simulink model "dIPC"  (R2014b)
settings: Solver=ode8  SolverMode=SingleTasking  StartTime=0.0  StopTime=3  FixedStep=1e-3  RelTol=1e-3
values from neighbouring files (symbols this model uses):
  deltav = 500    [DIPCRTinit.m]
  dv = 1500    [DIPCRTinit.m]
  g = [0;0;0]    [DIPCRTinit.m]
  j0 = 0.2    [DIPCRTinit.m]
  j1 = 0.5    [DIPCRTinit.m]
  j2 = 0.5    [DIPCRTinit.m]
  j3 = 0.5    [DIPCRTinit.m]
  j4 = 0.5    [DIPCRTinit.m]
  jv = 0.2    [DIPCRTinit.m]
  kappas = ks/20    (= 6)    [DIPCRTinit.m]
  kappav = 400    [DIPCRTinit.m]
  ks = 120    [DIPCRTinit.m]
  kv = 700    [DIPCRTinit.m]
  m0 = 1.4    [DIPCRTinit.m]
  m1 = 10    [DIPCRTinit.m]
  m2 = 10    [DIPCRTinit.m]
  m3 = 10    [DIPCRTinit.m]
  m4 = 10    [DIPCRTinit.m]
  mv = 1.4    [DIPCRTinit.m]
libraries: aerolibutil x16, dspinverses x3, aerolibtransform2 x2, simulink x2
settings Model: Creator=Martin  LastModifiedBy=Martin
settings OptimizationCC: BlockReduction=off  BooleanDataType=off  UseDivisionForNetSlopeComputation=off  OptimizeBlockIOStorage=off  BufferReuse=off  GlobalBufferReuse=off  ExpressionFolding=off  LocalBlockOutputs=off  SimCompilerOptimization=off
settings DebuggingCC: SaveWithParameterizedLinksMsg=none  UnderspecifiedInitializationDetection=Classic  MergeDetectMultiDrivingBlocksExec=none  SignalResolutionControl=TryResolveAllWithWarning  SolverPrmCheckMsg=none  FrameProcessingCompatibilityMsg=error
settings HardwareCC: TargetUnknown=on
settings RTWCC: RTWCompilerOptimization=off

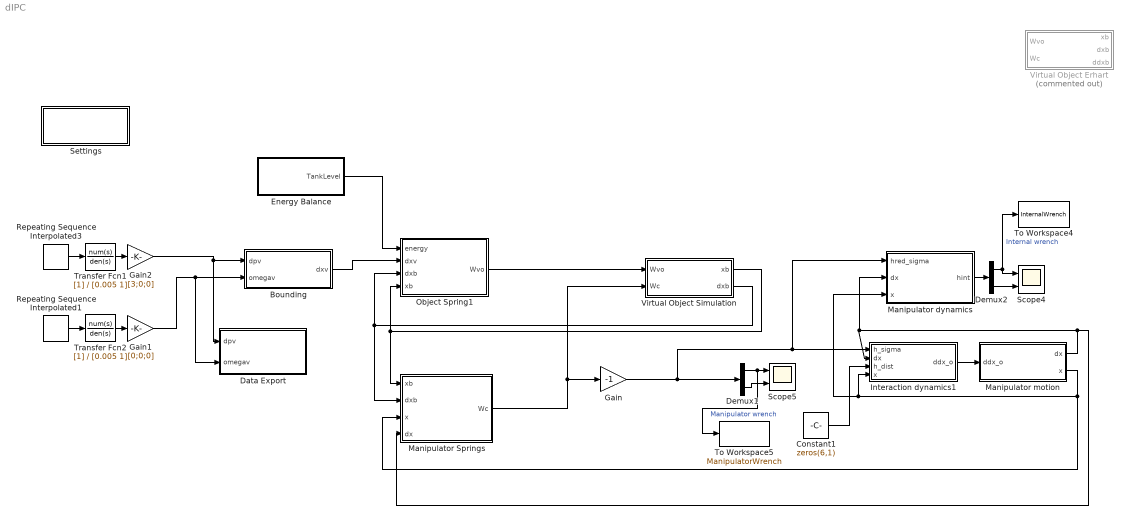
== system dIPC ==
  Bounding : Subsystem
  Constant1 : Constant  Value=zeros(6,1)
  Data Export : Subsystem
  Demux1 : Demux  Outputs=2
  Demux2 : Demux  Outputs=2
  Energy Balance : Subsystem
  Gain : Gain  Gain=-1
  Gain1 : Gain  Gain=[0;0;0]
  Gain2 : Gain  Gain=[3;0;0]
  Interaction dynamics1 : Subsystem
  Manipulator Springs : Subsystem
  Manipulator dynamics : Subsystem
  Manipulator motion : Subsystem
  Object Spring1 : Subsystem
  Repeating Sequence Interpolated1 : simulink/Sources/Repeating Sequence Interpolated  OutValues="[0 0 0.2 0, 0 0.5 0, 0  -0.4 0, 0 0.15 0, 0].'"  TimeValues=[0 0.1 0.25 0.4, 0.6 1 1.5, 1.7 2 2.3, 2.5 2.7 2.9, 3].'  LookUpMeth=Interpolation-Use End Values  tsamp=0.001  OutMin=[]  OutMax=[]  OutDataTypeStr=double  OutputDataTypeScalingMode=double  OutDataType=fixdt(0,8)  OutScaling=2^-10
  Repeating Sequence Interpolated3 : simulink/Sources/Repeating Sequence Interpolated  OutValues="[0 0 0.2 0, 0 0.5 0, 0  -0.4 0, 0 0.15 0, 0].'"  TimeValues=[0 0.1 0.25 0.4, 0.6 1 1.5, 1.7 2 2.3, 2.5 2.7 2.9, 3].'  LookUpMeth=Interpolation-Use End Values  tsamp=0.001  OutMin=[]  OutMax=[]  OutDataTypeStr=double  OutputDataTypeScalingMode=double  OutDataType=fixdt(0,8)  OutScaling=2^-10
  Scope4 : Scope  NumInputPorts=2
      settings: ShowLegends=on  YMin=-0.25~-0.25  YMax=0.25~0.25  SaveName=ScopeData6
  Scope5 : Scope  NumInputPorts=2
      settings: ShowLegends=on  TimeRange=3  YMin=-17.5~-15  YMax=12.5~17.5  SaveName=ScopeData11
  Settings : Subsystem
  To Workspace4 : ToWorkspace  VariableName=InternalWrench  SaveFormat=Timeseries  SampleTime=-1
  To Workspace5 : ToWorkspace  VariableName=ManipulatorWrench  SaveFormat=Timeseries  SampleTime=-1
  Transfer Fcn1 : TransferFcn  Denominator=[0.005 1]
  Transfer Fcn2 : TransferFcn  Denominator=[0.005 1]
  Virtual Object Erhart : Subsystem  Commented=on
  Virtual Object Simulation : Subsystem
  wires:
  Object Spring1/1(Wvo) -> Virtual Object Simulation/1(Wvo)
  Virtual Object Simulation/1(xb) -> Manipulator Springs/1(xb), Object Spring1/4(xb)
  Interaction dynamics1/1(ddx_o) -> Manipulator motion/1(ddx_o)
  Constant1/1 -> Interaction dynamics1/3(h_dist)
  Manipulator motion/2(x) -> Manipulator Springs/3(x), Manipulator dynamics/3(x), Interaction dynamics1/4(x)
  Virtual Object Simulation/2(dxb) -> Manipulator Springs/2(dxb), Object Spring1/3(dxb)
  Manipulator dynamics/1(hint) -> Demux2/1
  Demux2/2 -> Scope4/2
  Demux2/1 -> Scope4/1, To Workspace4/1  "Internal wrench"
  Repeating Sequence Interpolated3/1 -> Transfer Fcn1/1
  Transfer Fcn1/1 -> Gain2/1
  Transfer Fcn2/1 -> Gain1/1
  Demux1/2 -> Scope5/2
  Demux1/1 -> To Workspace5/1, Scope5/1  "Manipulator wrench"
  Gain1/1 -> Data Export/2(omegav), Bounding/2(omegav)
  Gain2/1 -> Data Export/1(dpv), Bounding/1(dpv)
  Bounding/1(dxv) -> Object Spring1/2(dxv)
  Repeating Sequence Interpolated1/1 -> Transfer Fcn2/1
  Manipulator Springs/1(Wc) -> Virtual Object Simulation/2(Wc), Gain/1
  Gain/1 -> Manipulator dynamics/1(hred_sigma), Interaction dynamics1/1(h_sigma), Demux1/1
  Manipulator motion/1(dx) -> Manipulator Springs/4(dx), Manipulator dynamics/2(dx), Interaction dynamics1/2(dx)
  Energy Balance/1(TankLevel) -> Object Spring1/1(energy)

== system dIPC/Bounding ==
  dpv : Inport
  omegav : Inport  Port=2
  Mux : Mux  Inputs=2
  dxv : Outport
  wires:
  dpv/1 -> Mux/1
  omegav/1 -> Mux/2
  Mux/1 -> dxv/1

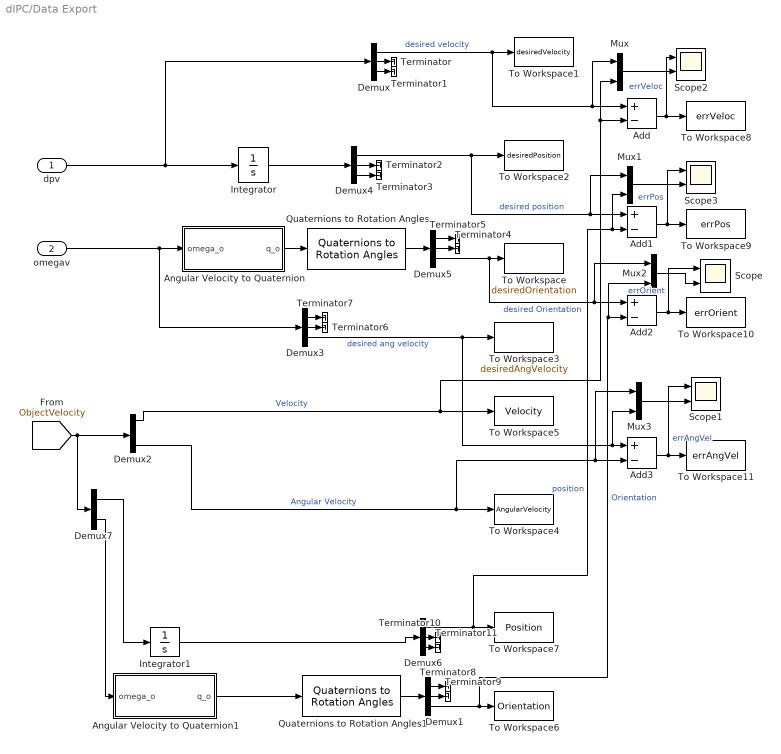
== system dIPC/Data Export ==
  dpv : Inport
  omegav : Inport  Port=2
  Add{,1..3} (4 alike) : Sum  Inputs=+-
  Angular Velocity to Quaternion : Subsystem
  Angular Velocity to Quaternion1 : Subsystem
  Demux{,1,3..6} (6 alike) : Demux  Outputs=3
  Demux2 : Demux  Outputs=6
  Demux7 : Demux  Outputs=2
  Integrator : Integrator
  Integrator1 : Integrator  InitialCondition=[0 0 0]'
  Mux{,1..3} (4 alike) : Mux  Inputs=2
  Quaternions to Rotation Angles : aerolibtransform2/Quaternions to Rotation Angles  rotationOrder=XYZ
  Quaternions to Rotation Angles1 : aerolibtransform2/Quaternions to Rotation Angles  rotationOrder=XYZ
  Scope{,1..3} (4 alike) : Scope  NumInputPorts=2
      Scope settings: YMin=-0.03~-0  YMax=0.035~0.275  SaveName=ScopeData13
      Scope1 settings: ShowLegends=on  YMin=-0.1~-0.4  YMax=0.1~0.6  SaveName=ScopeData37
      Scope2 settings: ShowLegends=on  TimeRange=3  YMin=-0.6~-1.5  YMax=0.6~1.5  SaveName=ScopeData19
      Scope3 settings: YMin=-0.0025~0  YMax=0.03~0.13  SaveName=ScopeData39
  Terminator{,1..11} (12 alike) : Terminator
  To Workspace : ToWorkspace  VariableName=desiredOrientation  SaveFormat=Timeseries  SampleTime=-1
  To Workspace1 : ToWorkspace  VariableName=desiredVelocity  SaveFormat=Timeseries  SampleTime=-1
  To Workspace10 : ToWorkspace  VariableName=errOrient  SaveFormat=Timeseries  SampleTime=-1
  To Workspace11 : ToWorkspace  VariableName=errAngVel  SaveFormat=Timeseries  SampleTime=-1
  To Workspace2 : ToWorkspace  VariableName=desiredPosition  SaveFormat=Timeseries  SampleTime=-1
  To Workspace3 : ToWorkspace  VariableName=desiredAngVelocity  SaveFormat=Timeseries  SampleTime=-1
  To Workspace4 : ToWorkspace  VariableName=AngularVelocity  SaveFormat=Timeseries  SampleTime=-1
  To Workspace5 : ToWorkspace  VariableName=Velocity  SaveFormat=Timeseries  SampleTime=-1
  To Workspace6 : ToWorkspace  VariableName=Orientation  SaveFormat=Timeseries  SampleTime=-1
  To Workspace7 : ToWorkspace  VariableName=Position  SaveFormat=Timeseries  SampleTime=-1
  To Workspace8 : ToWorkspace  VariableName=errVeloc  SaveFormat=Timeseries  SampleTime=-1
  To Workspace9 : ToWorkspace  VariableName=errPos  SaveFormat=Timeseries  SampleTime=-1
  wires:
  Demux4/1 -> Mux1/1, Add1/1, To Workspace2/1  "desired position"
  Demux/1 -> Mux/1, Add/1, To Workspace1/1  "desired velocity"
  Integrator/1 -> Demux4/1
  dpv/1 -> Demux/1, Integrator/1
  Demux/2 -> Terminator/1
  Demux/3 -> Terminator1/1
  Demux4/2 -> Terminator2/1
  Demux4/3 -> Terminator3/1
  Quaternions to Rotation Angles/1 -> Demux5/1
  Demux5/3 -> Mux2/1, Add2/1, To Workspace/1  "desired Orientation"
  Demux3/3 -> Mux3/2, Add3/1, To Workspace3/1  "desired ang velocity"
  Angular Velocity to Quaternion/1(q_o) -> Quaternions to Rotation Angles/1
  omegav/1 -> Demux3/1, Angular Velocity to Quaternion/1(omega_o)
  Demux5/2 -> Terminator4/1
  Demux5/1 -> Terminator5/1
  Demux3/2 -> Terminator6/1
  Demux3/1 -> Terminator7/1
  Demux2/1 -> Mux/2, Add/2, To Workspace5/1  "Velocity"
  Demux2/6 -> Mux3/1, Add3/2, To Workspace4/1  "Angular Velocity"
  [ObjectVelocity] -> Demux7/1, Demux2/1
  Quaternions to Rotation Angles1/1 -> Demux1/1
  Demux1/3 -> Mux2/2, Add2/2, To Workspace6/1  "Orientation"
  Demux1/2 -> Terminator9/1
  Demux1/1 -> Terminator8/1
  Demux6/1 -> Mux1/2, Add1/2, To Workspace7/1  "position"
  Demux6/2 -> Terminator10/1
  Demux6/3 -> Terminator11/1
  Demux7/1 -> Integrator1/1
  Integrator1/1 -> Demux6/1
  Demux7/2 -> Angular Velocity to Quaternion1/1(omega_o)
  Angular Velocity to Quaternion1/1(q_o) -> Quaternions to Rotation Angles1/1
  Add/1 -> Scope2/1, To Workspace8/1  "errVeloc"
  Add1/1 -> Scope3/1, To Workspace9/1  "errPos"
  Add2/1 -> Scope/1, To Workspace10/1  "errOrient"
  Add3/1 -> Scope1/1, To Workspace11/1  "errAngVel"
  Mux/1 -> Scope2/2
  Mux1/1 -> Scope3/2
  Mux2/1 -> Scope/2
  Mux3/1 -> Scope1/2

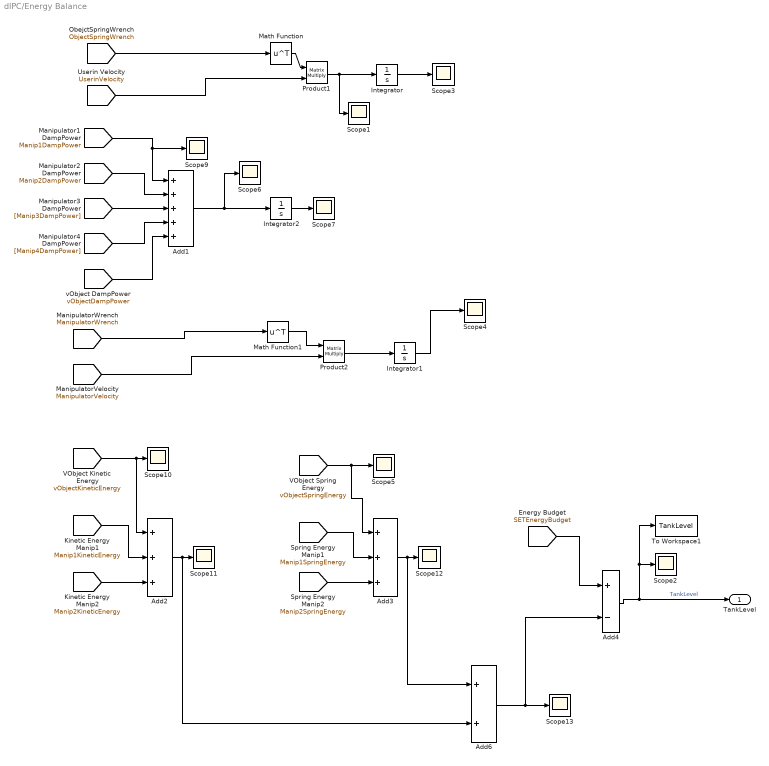
== system dIPC/Energy Balance ==
  Add1 : Sum  Inputs=+++++
  Add2 : Sum  Inputs=+++
  Add3 : Sum  Inputs=+++
  Add4 : Sum  Inputs=+-
  Add6 : Sum
  Integrator : Integrator
  Integrator1 : Integrator
  Integrator2 : Integrator
  Math Function : Math  Operator=transpose  SaturateOnIntegerOverflow=on
  Math Function1 : Math  Operator=transpose  SaturateOnIntegerOverflow=on
  Product1 : Product  Multiplication=Matrix(*)
  Product2 : Product  Multiplication=Matrix(*)
  Scope{1..7,9..13} (12 alike) : Scope
      Scope1 settings: YMin=0  YMax=60  SaveName=ScopeData5
      Scope10 settings: YMin=0  YMax=0.5  SaveName=ScopeData3
      Scope11 settings: YMin=0  YMax=25  SaveName=ScopeData23
      Scope12 settings: YMin=0  YMax=0.6  SaveName=ScopeData36
      Scope13 settings: YMin=1  YMax=9  SaveName=ScopeData38
      Scope2 settings: TimeRange=4.999  YMin=0  YMax=10
      Scope3 settings: TimeRange=5  YMin=0  YMax=12  SaveName=ScopeData14
      Scope4 settings: YMin=-60  YMax=10  SaveName=ScopeData12
      Scope5 settings: YMin=-4.16334e-17  YMax=0.575  SaveName=ScopeData42
      Scope6 settings: YMin=-0.3  YMax=0.05  SaveName=ScopeData40
      Scope7 settings: YMin=675  YMax=1000  SaveName=ScopeData41
      Scope9 settings: YMin=0  YMax=3e-05  SaveName=ScopeData46
  To Workspace1 : ToWorkspace  VariableName=TankLevel  SaveFormat=Timeseries  SampleTime=-1
  TankLevel : Outport
  wires:
  Add4/1 -> TankLevel/1, To Workspace1/1, Scope2/1  "TankLevel"
  Product1/1 -> Integrator/1, Scope1/1
  [UserinVelocity] -> Product1/2
  Integrator/1 -> Scope3/1
  [Manip1DampPower] -> Scope9/1, Add1/1
  [Manip2DampPower] -> Add1/2
  [Manip3DampPower] -> Add1/3
  [Manip4DampPower] -> Add1/4
  [vObjectDampPower] -> Add1/5
  Add1/1 -> Integrator2/1, Scope6/1
  Integrator2/1 -> Scope7/1
  Math Function/1 -> Product1/1
  [ObjectSpringWrench] -> Math Function/1
  Add6/1 -> Add4/2, Scope13/1
  Product2/1 -> Integrator1/1
  Math Function1/1 -> Product2/1
  [ManipulatorVelocity] -> Product2/2
  [ManipulatorWrench] -> Math Function1/1
  Integrator1/1 -> Scope4/1
  [SETEnergyBudget] -> Add4/1
  [vObjectSpringEnergy] -> Scope5/1, Add3/1
  [vObjectKineticEnergy] -> Add2/1, Scope10/1
  Add2/1 -> Add6/2, Scope11/1
  Add3/1 -> Add6/1, Scope12/1
  [Manip2SpringEnergy] -> Add3/3
  [Manip1SpringEnergy] -> Add3/2
  [Manip2KineticEnergy] -> Add2/3
  [Manip1KineticEnergy] -> Add2/2

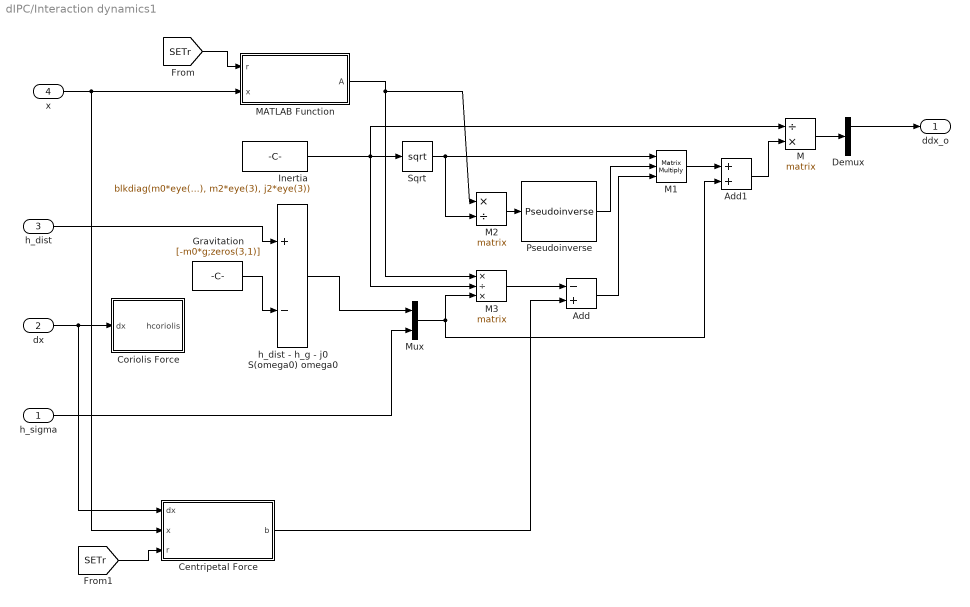
== system dIPC/Interaction dynamics1 ==
  h_sigma : Inport
  dx : Inport  Port=2
  h_dist : Inport  Port=3
  x : Inport  Port=4
  Add : Sum  Inputs=-+
  Add1 : Sum
  Centripetal Force : MATLAB Function  TreatAsAtomicUnit=on
  Coriolis Force : MATLAB Function  TreatAsAtomicUnit=on
  Demux : Demux  Outputs=3
  Gravitation : Constant  Value=[-m0*g;zeros(3,1)]
  Inertia : Constant  Value=blkdiag(m0*eye(3),j0*eye(3),m1*eye(3), j1*eye(3), m2*eye(3), j2*eye(3))
  M : Product  Inputs=/*  Multiplication=Matrix(*)
  M1 : Product  Inputs=***  Multiplication=Matrix(*)
  M2 : Product  Inputs=*/  Multiplication=Matrix(*)
  M3 : Product  Inputs=*/*  Multiplication=Matrix(*)
  MATLAB Function : MATLAB Function  TreatAsAtomicUnit=on
  Mux : Mux  Inputs=2
  Pseudoinverse : dspinverses/Pseudoinverse  wanterr=off
  Sqrt : Sqrt  SaturateOnIntegerOverflow=on
  "h_dist - h_g - j0 S(omega0) omega0 " : Sum  Inputs=+-
  ddx_o : Outport
  wires:
  h_dist/1 -> "h_dist - h_g - j0 S(omega0) omega0 "/1
  Gravitation/1 -> "h_dist - h_g - j0 S(omega0) omega0 "/2
  dx/1 -> Centripetal Force/1(dx), Coriolis Force/1(dx)
  x/1 -> MATLAB Function/2(x), Centripetal Force/2(x)
  Inertia/1 -> M/1, M3/2, Sqrt/1
  Sqrt/1 -> M2/2, M1/1
  MATLAB Function/1(A) -> M3/1, M2/1
  M2/1 -> Pseudoinverse/1
  Pseudoinverse/1 -> M1/2
  Add/1 -> M1/3
  Centripetal Force/1(b) -> Add/2
  M3/1 -> Add/1
  Mux/1 -> Add1/2, M3/3
  "h_dist - h_g - j0 S(omega0) omega0 "/1 -> Mux/1
  h_sigma/1 -> Mux/2
  M/1 -> Demux/1
  Demux/1 -> ddx_o/1
  M1/1 -> Add1/1
  Add1/1 -> M/2
  [SETr] -> MATLAB Function/1(r)
  [SETr] -> Centripetal Force/3(r)

== system dIPC/Manipulator Springs ==
  xb : Inport
  dxb : Inport  Port=2
  x : Inport  Port=3
  dx : Inport  Port=4
  Demux1 : Demux  Outputs=2
  Demux2 : Demux  Outputs=2
  Demux3 : Demux  Outputs=2
  Grasp Matrix : MATLAB Function  TreatAsAtomicUnit=on
  Math Function : Math  Operator=transpose  SaturateOnIntegerOverflow=on
  Mux : Mux  Inputs=2
  Product : Product  Multiplication=Matrix(*)
  Spring 1 : Subsystem
  Spring 2 : Subsystem
  Wc : Outport
  tag scope: ManipulatorWrench=global
  wires:
  Spring 2/1(Wc2) -> Mux/2
  Mux/1 -> [ManipulatorWrench], Wc/1
  Grasp Matrix/1(G) -> Math Function/1
  Math Function/1 -> Product/1
  dxb/1 -> Product/2
  Product/1 -> Demux3/1
  xb/1 -> Spring 1/1(xb), Spring 2/1(xb), Grasp Matrix/1(x)
  Demux3/2 -> Spring 2/2(dxb2)
  Demux3/1 -> Spring 1/2(dxb1)
  Spring 1/1(Wc1) -> Mux/1
  Demux2/1 -> Spring 1/3(x1)
  Demux2/2 -> Spring 2/3(x2)
  Demux1/1 -> Spring 1/4(dx1)
  Demux1/2 -> Spring 2/4(dx2)
  dx/1 -> Demux1/1
  x/1 -> Demux2/1
  [SETrv] -> Grasp Matrix/2(rv)

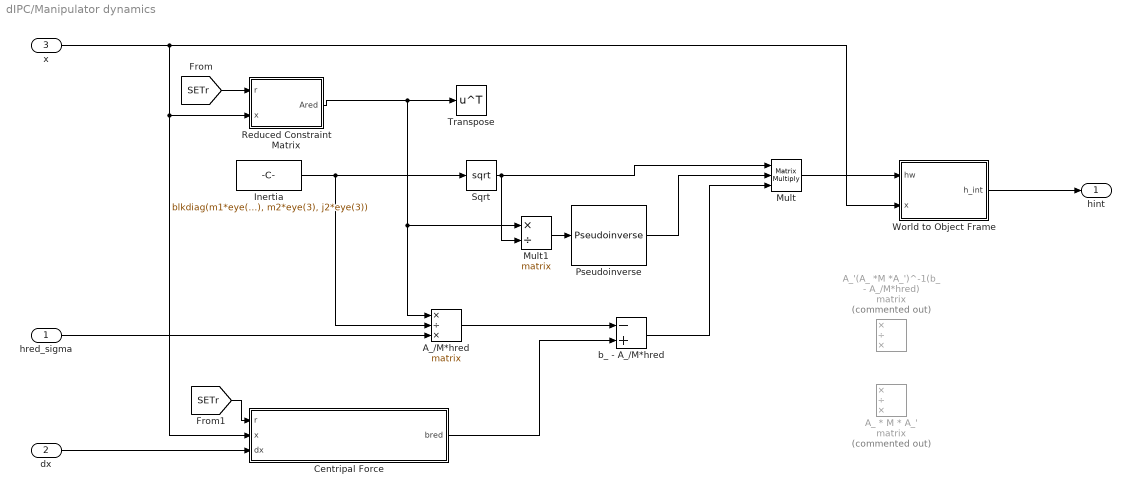
== system dIPC/Manipulator dynamics ==
  hred_sigma : Inport
  dx : Inport  Port=2
  x : Inport  Port=3
  A_ * M * A_' : Product  Commented=on  Inputs=*/*  Multiplication=Matrix(*)
  A_'(A_ *M *A_')^-1(b_ - A_/M*hred) : Product  Commented=on  Inputs=*/*  Multiplication=Matrix(*)
  A_/M*hred : Product  Inputs=*/*  Multiplication=Matrix(*)
  Centripal Force : MATLAB Function  TreatAsAtomicUnit=on
  Inertia : Constant  Value=blkdiag(m1*eye(3), j1*eye(3), m2*eye(3), j2*eye(3))
  Mult : Product  Inputs=***  Multiplication=Matrix(*)
  Mult1 : Product  Inputs=*/  Multiplication=Matrix(*)
  Pseudoinverse : dspinverses/Pseudoinverse  wanterr=off
  Reduced Constraint Matrix : MATLAB Function  TreatAsAtomicUnit=on
  Sqrt : Sqrt  SaturateOnIntegerOverflow=on
  Transpose : Math  Operator=transpose  SaturateOnIntegerOverflow=on
  World to Object Frame : MATLAB Function  TreatAsAtomicUnit=on
  b_ - A_/M*hred : Sum  Inputs=-+
  hint : Outport
  wires:
  Reduced Constraint Matrix/1(Ared) -> Transpose/1, A_/M*hred/1, Mult1/1
  Inertia/1 -> Sqrt/1, A_/M*hred/2
  dx/1 -> Centripal Force/3(dx)
  A_/M*hred/1 -> b_ - A_/M*hred/1
  hred_sigma/1 -> A_/M*hred/3
  World to Object Frame/1(h_int) -> hint/1
  x/1 -> Centripal Force/2(x), Reduced Constraint Matrix/2(x), World to Object Frame/2(x)
  Centripal Force/1(bred) -> b_ - A_/M*hred/2
  Mult/1 -> World to Object Frame/1(hw)
  b_ - A_/M*hred/1 -> Mult/3
  Sqrt/1 -> Mult1/2, Mult/1
  Mult1/1 -> Pseudoinverse/1
  Pseudoinverse/1 -> Mult/2
  [SETr] -> Reduced Constraint Matrix/1(r)
  [SETr] -> Centripal Force/1(r)

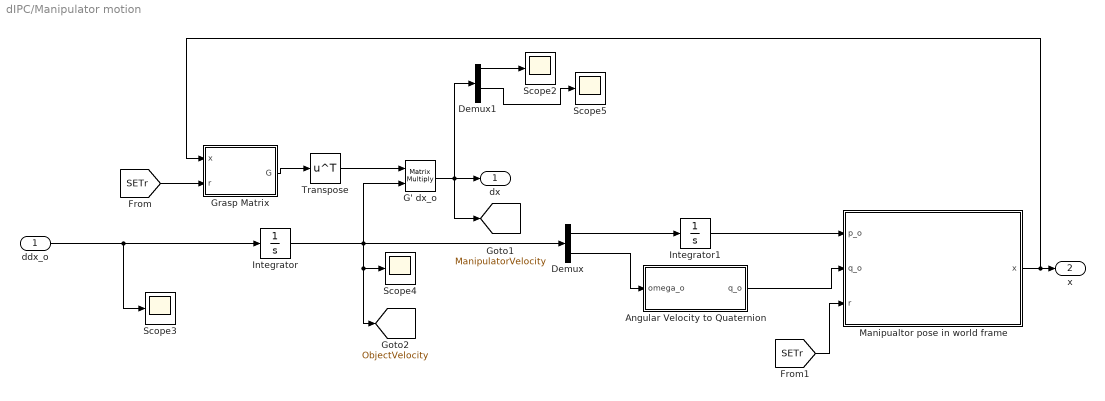
== system dIPC/Manipulator motion ==
  ddx_o : Inport
  Angular Velocity to Quaternion : Subsystem
  Demux : Demux  Outputs=2
  Demux1 : Demux
  G' dx_o : Product  Multiplication=Matrix(*)
  Grasp Matrix : MATLAB Function  TreatAsAtomicUnit=on
  Integrator : Integrator  InitialCondition=zeros(6,1)
  Integrator1 : Integrator  InitialCondition=[0 0 0]'
  Manipualtor pose in world frame : MATLAB Function  TreatAsAtomicUnit=on
  Scope{2..5} (4 alike) : Scope
      Scope2 settings: YMin=-0.02  YMax=0.16  SaveName=ScopeData12
      Scope3 settings: SaveName=ScopeData7
      Scope4 settings: SaveName=ScopeData16
      Scope5 settings: ShowLegends=on  YMin=-0.4  YMax=0.5  SaveName=ScopeData40
  Transpose : Math  Operator=transpose  SaturateOnIntegerOverflow=on
  dx : Outport
  x : Outport  Port=2
  tag scope: ManipulatorVelocity=global, ObjectVelocity=global
  wires:
  ddx_o/1 -> Scope3/1, Integrator/1
  Integrator/1 -> Scope4/1, [ObjectVelocity], G' dx_o/2, Demux/1
  Grasp Matrix/1(G) -> Transpose/1
  Transpose/1 -> G' dx_o/1
  G' dx_o/1 -> [ManipulatorVelocity], Demux1/1, dx/1
  Demux/2 -> Angular Velocity to Quaternion/1(omega_o)
  Demux/1 -> Integrator1/1
  Integrator1/1 -> Manipualtor pose in world frame/1(p_o)
  Manipualtor pose in world frame/1(x) -> Grasp Matrix/1(x), x/1
  Angular Velocity to Quaternion/1(q_o) -> Manipualtor pose in world frame/2(q_o)
  Demux1/1 -> Scope2/1
  Demux1/3 -> Scope5/1
  [SETr] -> Grasp Matrix/2(r)
  [SETr] -> Manipualtor pose in world frame/3(r)

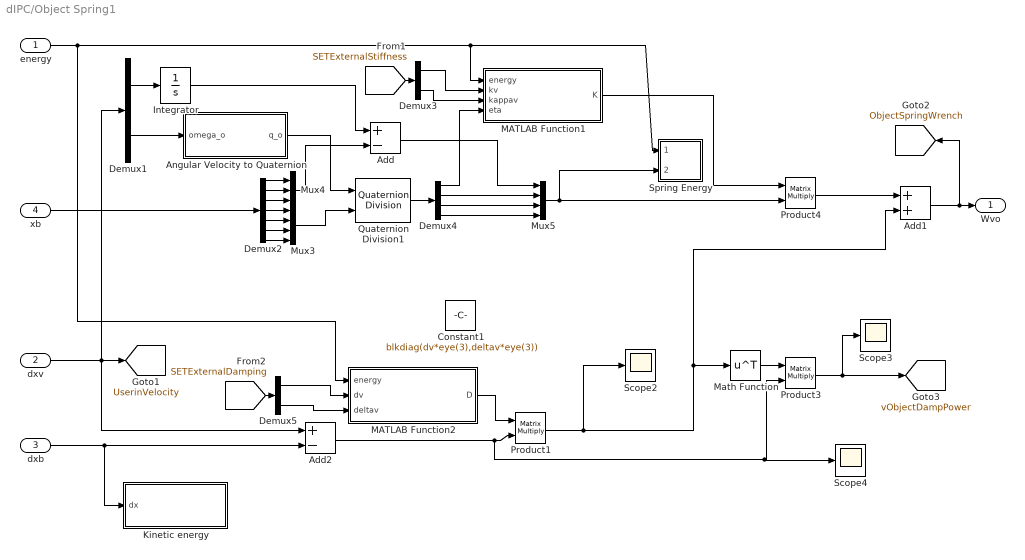
== system dIPC/Object Spring1 ==
  energy : Inport
  dxv : Inport  Port=2
  dxb : Inport  Port=3
  xb : Inport  Port=4
  Add : Sum  Inputs=+-
  Add1 : Sum
  Add2 : Sum  Inputs=+-
  Angular Velocity to Quaternion : Subsystem
  Constant1 : Constant  Value=blkdiag(dv*eye(3),deltav*eye(3))
  Demux1 : Demux  Outputs=2
  Demux2 : Demux  Outputs=7
  Demux3 : Demux  Outputs=2
  Demux4 : Demux
  Demux5 : Demux  Outputs=2
  Integrator : Integrator
  Kinetic energy : Subsystem
  MATLAB Function1 : MATLAB Function  TreatAsAtomicUnit=on
  MATLAB Function2 : MATLAB Function  TreatAsAtomicUnit=on
  Math Function : Math  Operator=transpose  SaturateOnIntegerOverflow=on
  Mux3 : Mux
  Mux4 : Mux  Inputs=3
  Mux5 : Mux
  Product1 : Product  Multiplication=Matrix(*)
  Product3 : Product  Multiplication=Matrix(*)
  Product4 : Product  Multiplication=Matrix(*)
  Quaternion Division1 : aerolibutil/Quaternion Division
  Scope2 : Scope
      settings: YMin=-1500  YMax=6500  SaveName=ScopeData4
  Scope3 : Scope
      settings: YMin=0  YMax=8500  SaveName=ScopeData2
  Scope4 : Scope
      settings: YMin=-3.5  YMax=3  SaveName=ScopeData35
  Spring Energy : Subsystem
  Wvo : Outport
  tag scope: ObjectSpringWrench=global, UserinVelocity=global, vObjectDampPower=global
  wires:
  Add1/1 -> Wvo/1, [ObjectSpringWrench]
  Product4/1 -> Add1/1
  Product1/1 -> Scope2/1, Math Function/1, Add1/2
  MATLAB Function1/1(K) -> Product4/1
  Demux4/1 -> MATLAB Function1/4(eta)
  Add/1 -> Mux5/1
  Demux4/2 -> Mux5/2
  Demux4/3 -> Mux5/3
  Demux4/4 -> Mux5/4
  Quaternion Division1/1 -> Demux4/1
  xb/1 -> Demux2/1
  Demux2/4 -> Mux3/1
  Demux2/5 -> Mux3/2
  Demux2/6 -> Mux3/3
  Demux2/7 -> Mux3/4
  Demux2/1 -> Mux4/1
  Demux2/2 -> Mux4/2
  Demux2/3 -> Mux4/3
  Mux4/1 -> Add/2
  Mux3/1 -> Quaternion Division1/2
  Add2/1 -> Scope4/1, Product3/2, Product1/2
  dxv/1 -> [UserinVelocity], Add2/1, Demux1/1
  dxb/1 -> Kinetic energy/1(dx), Add2/2
  Product3/1 -> Scope3/1, [vObjectDampPower]
  Math Function/1 -> Product3/1
  Mux5/1 -> Spring Energy/2(deltax), Product4/2
  Demux1/1 -> Integrator/1
  Integrator/1 -> Add/1
  Demux1/2 -> Angular Velocity to Quaternion/1(omega_o)
  Angular Velocity to Quaternion/1(q_o) -> Quaternion Division1/1
  energy/1 -> MATLAB Function1/1(energy), Spring Energy/1(energy), MATLAB Function2/1(energy)
  MATLAB Function2/1(D) -> Product1/1
  [SETExternalStiffness] -> Demux3/1
  Demux3/1 -> MATLAB Function1/2(kv)
  Demux3/2 -> MATLAB Function1/3(kappav)
  [SETExternalDamping] -> Demux5/1
  Demux5/2 -> MATLAB Function2/3(deltav)
  Demux5/1 -> MATLAB Function2/2(dv)

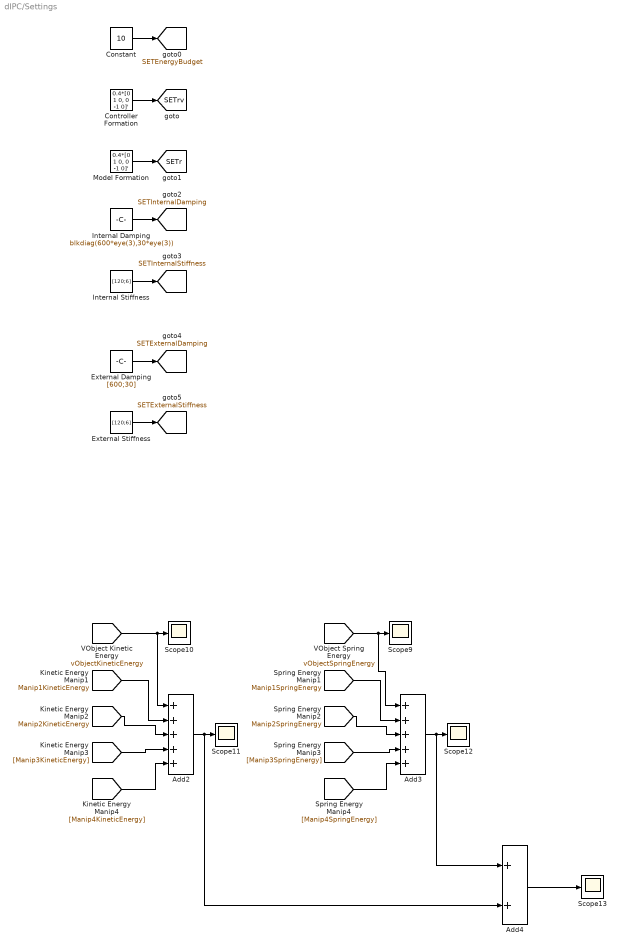
== system dIPC/Settings ==
  Add2 : Sum  Inputs=+++++
  Add3 : Sum  Inputs=+++++
  Add4 : Sum
  Constant : Constant  Value=10
  Controller Formation : Constant  Value=0.4*[0 1 0, 0 -1 0]'
  External Damping : Constant  Value=[600;30]
  External Stiffness : Constant  Value=[120;6]
  Internal Damping : Constant  Value=blkdiag(600*eye(3),30*eye(3))
  Internal Stiffness : Constant  Value=[120;6]
  Model Formation : Constant  Value=0.4*[0 1 0, 0 -1 0]'
  Scope{9..13} (5 alike) : Scope
      Scope10 settings: YMin=0  YMax=0.5  SaveName=ScopeData29
      Scope11 settings: YMin=0  YMax=25  SaveName=ScopeData30
      Scope12 settings: YMin=0  YMax=0.6  SaveName=ScopeData31
      Scope13 settings: YMin=0  YMax=50  SaveName=ScopeData32
      Scope9 settings: YMin=-4.16334e-17  YMax=0.575  SaveName=ScopeData28
  tag scope: SETEnergyBudget=global, SETExternalDamping=global, SETExternalStiffness=global, SETInternalDamping=global, SETInternalStiffness=global, SETr=global, SETrv=global
  wires:
  [vObjectSpringEnergy] -> Add3/1, Scope9/1
  [vObjectKineticEnergy] -> Add2/1, Scope10/1
  Add2/1 -> Add4/2, Scope11/1
  Add3/1 -> Add4/1, Scope12/1
  Add4/1 -> Scope13/1
  [Manip4KineticEnergy] -> Add2/5
  [Manip4SpringEnergy] -> Add3/5
  [Manip3SpringEnergy] -> Add3/4
  [Manip2SpringEnergy] -> Add3/3
  [Manip1SpringEnergy] -> Add3/2
  [Manip3KineticEnergy] -> Add2/4
  [Manip2KineticEnergy] -> Add2/3
  [Manip1KineticEnergy] -> Add2/2
  Constant/1 -> [SETEnergyBudget]
  Model Formation/1 -> [SETr]
  Controller Formation/1 -> [SETrv]
  Internal Damping/1 -> [SETInternalDamping]
  Internal Stiffness/1 -> [SETInternalStiffness]
  External Damping/1 -> [SETExternalDamping]
  External Stiffness/1 -> [SETExternalStiffness]

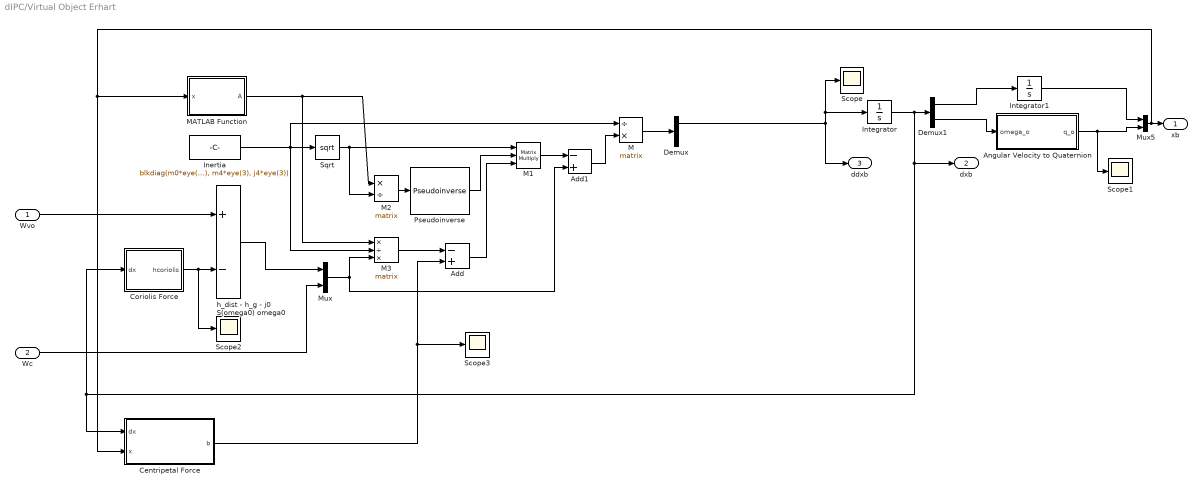
== system dIPC/Virtual Object Erhart ==
  Wvo : Inport
  Wc : Inport  Port=2
  Add : Sum  Inputs=-+
  Add1 : Sum  Inputs=-+
  Angular Velocity to Quaternion : Subsystem
  Centripetal Force : MATLAB Function  TreatAsAtomicUnit=on
  Coriolis Force : MATLAB Function  TreatAsAtomicUnit=on
  Demux : Demux  Outputs=5
  Demux1 : Demux  Outputs=2
  Inertia : Constant  Value=blkdiag(m0*eye(3),j0*eye(3),m1*eye(3), j1*eye(3), m2*eye(3), j2*eye(3),m3*eye(3), j3*eye(3), m4*eye(3), j4*eye(3))
  Integrator : Integrator  InitialCondition=zeros(6,1)
  Integrator1 : Integrator  InitialCondition=[0 0 0]'
  M : Product  Inputs=/*  Multiplication=Matrix(*)
  M1 : Product  Inputs=***  Multiplication=Matrix(*)
  M2 : Product  Inputs=*/  Multiplication=Matrix(*)
  M3 : Product  Inputs=*/*  Multiplication=Matrix(*)
  MATLAB Function : MATLAB Function  TreatAsAtomicUnit=on
  Mux : Mux  Inputs=2
  Mux5 : Mux  Inputs=2
  Pseudoinverse : dspinverses/Pseudoinverse  wanterr=off
  Scope{,1..3} (4 alike) : Scope
      Scope1 settings: SaveName=ScopeData8
      Scope2 settings: SaveName=ScopeData15
      Scope3 settings: YMin=-1  YMax=1  SaveName=ScopeData17
  Sqrt : Sqrt  SaturateOnIntegerOverflow=on
  "h_dist - h_g - j0 S(omega0) omega0 " : Sum  Inputs=+-
  xb : Outport
  dxb : Outport  Port=2
  ddxb : Outport  Port=3
  wires:
  Demux/1 -> Scope/1, Integrator/1, ddxb/1
  Integrator/1 -> Demux1/1, Coriolis Force/1(dx), Centripetal Force/1(dx), dxb/1
  Demux1/2 -> Angular Velocity to Quaternion/1(omega_o)
  Demux1/1 -> Integrator1/1
  Integrator1/1 -> Mux5/1
  Angular Velocity to Quaternion/1(q_o) -> Scope1/1, Mux5/2
  Wvo/1 -> "h_dist - h_g - j0 S(omega0) omega0 "/1
  Coriolis Force/1(hcoriolis) -> Scope2/1, "h_dist - h_g - j0 S(omega0) omega0 "/2
  Mux5/1 -> MATLAB Function/1(x), Centripetal Force/2(x), xb/1
  Inertia/1 -> M/1, M3/2, Sqrt/1
  Sqrt/1 -> M2/2, M1/1
  MATLAB Function/1(A) -> M3/1, M2/1
  M2/1 -> Pseudoinverse/1
  Pseudoinverse/1 -> M1/2
  Add/1 -> M1/3
  Centripetal Force/1(b) -> Scope3/1, Add/2
  M3/1 -> Add/1
  Mux/1 -> Add1/2, M3/3
  "h_dist - h_g - j0 S(omega0) omega0 "/1 -> Mux/1
  Wc/1 -> Mux/2
  M1/1 -> Add1/1
  Add1/1 -> M/2
  M/1 -> Demux/1

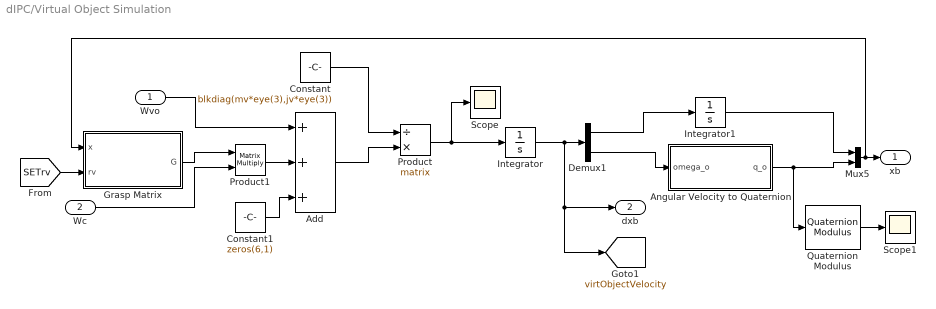
== system dIPC/Virtual Object Simulation ==
  Wvo : Inport
  Wc : Inport  Port=2
  Add : Sum  Inputs=+++
  Angular Velocity to Quaternion : Subsystem
  Constant : Constant  Value=blkdiag(mv*eye(3),jv*eye(3))
  Constant1 : Constant  Value=zeros(6,1)
  Demux1 : Demux  Outputs=2
  Grasp Matrix : MATLAB Function  TreatAsAtomicUnit=on
  Integrator : Integrator  InitialCondition=zeros(6,1)
  Integrator1 : Integrator  InitialCondition=[0 0 0]'
  Mux5 : Mux  Inputs=2
  Product : Product  Inputs=/*  Multiplication=Matrix(*)
  Product1 : Product  Inputs=**  Multiplication=Matrix(*)
  Quaternion Modulus : aerolibutil/Quaternion Modulus
  Scope : Scope
  Scope1 : Scope
      settings: TimeRange=3  YMin=1  YMax=1  SaveName=ScopeData34
  xb : Outport  PortDimensions=7
  dxb : Outport  Port=2
  tag scope: virtObjectVelocity=global
  wires:
  Add/1 -> Product/2
  Constant/1 -> Product/1
  Product/1 -> Scope/1, Integrator/1
  Integrator/1 -> Demux1/1, [virtObjectVelocity], dxb/1
  Demux1/2 -> Angular Velocity to Quaternion/1(omega_o)
  Demux1/1 -> Integrator1/1
  Integrator1/1 -> Mux5/1
  Angular Velocity to Quaternion/1(q_o) -> Quaternion Modulus/1, Mux5/2
  Mux5/1 -> Grasp Matrix/1(x), xb/1
  Wvo/1 -> Add/1
  Product1/1 -> Add/2
  Grasp Matrix/1(G) -> Product1/1
  Wc/1 -> Product1/2
  Quaternion Modulus/1 -> Scope1/1
  Constant1/1 -> Add/3
  [SETrv] -> Grasp Matrix/2(rv)

== system dIPC/Data Export/Angular Velocity to Quaternion ==
  omega_o : Inport
  Constant : Constant  Value=0
  Gain : Gain  Gain=0.5
  Integrator : Integrator  InitialCondition=[1; 0; 0; 0]
  Mux : Mux  Inputs=2
  Quaternion Multiplication : aerolibutil/Quaternion Multiplication
  Quaternion Normalize : aerolibutil/Quaternion Normalize
  Scope : Scope
      settings: ShowLegends=on  SaveName=ScopeData9
  q_o : Outport
  wires:
  omega_o/1 -> Gain/1
  Gain/1 -> Mux/2
  Constant/1 -> Mux/1
  Quaternion Multiplication/1 -> Integrator/1
  Integrator/1 -> Quaternion Normalize/1
  Mux/1 -> Quaternion Multiplication/1
  Quaternion Normalize/1 -> Quaternion Multiplication/2, q_o/1, Scope/1

== system dIPC/Data Export/Angular Velocity to Quaternion1 ==
  omega_o : Inport
  Constant : Constant  Value=0
  Gain : Gain  Gain=0.5
  Integrator : Integrator  InitialCondition=[1; 0; 0; 0]
  Mux : Mux  Inputs=2
  Quaternion Multiplication : aerolibutil/Quaternion Multiplication
  Quaternion Normalize : aerolibutil/Quaternion Normalize
  Scope : Scope
      settings: ShowLegends=on  SaveName=ScopeData9
  q_o : Outport
  wires:
  omega_o/1 -> Gain/1
  Gain/1 -> Mux/2
  Constant/1 -> Mux/1
  Integrator/1 -> Quaternion Normalize/1
  Mux/1 -> Quaternion Multiplication/1
  Quaternion Multiplication/1 -> Integrator/1
  Quaternion Normalize/1 -> Quaternion Multiplication/2, q_o/1, Scope/1

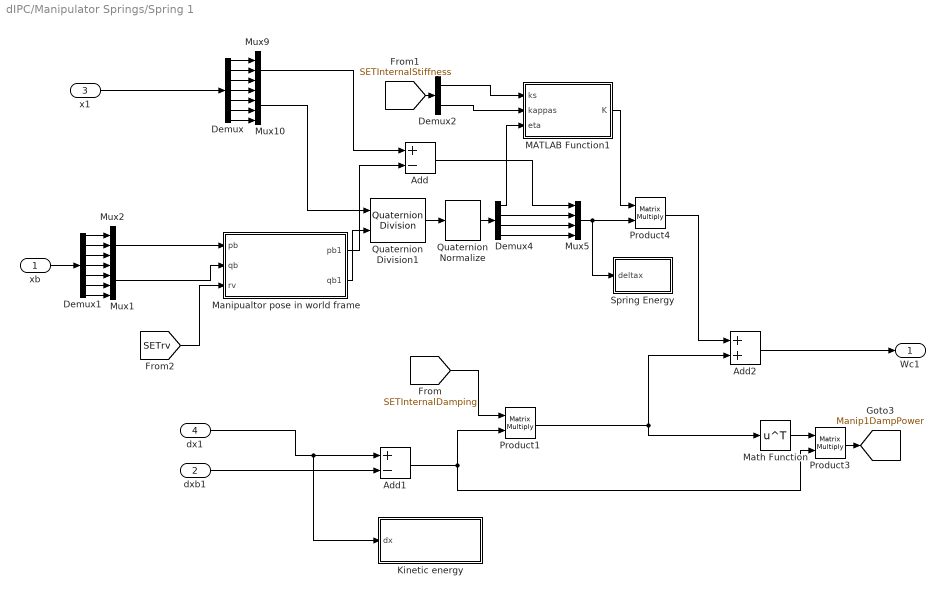
== system dIPC/Manipulator Springs/Spring 1 ==
  xb : Inport
  dxb1 : Inport  Port=2
  x1 : Inport  Port=3
  dx1 : Inport  Port=4
  Add : Sum  Inputs=+-
  Add1 : Sum  Inputs=+-
  Add2 : Sum
  Demux : Demux  Outputs=7
  Demux1 : Demux  Outputs=7
  Demux2 : Demux  Outputs=2
  Demux4 : Demux
  Kinetic energy : Subsystem
  MATLAB Function1 : MATLAB Function  TreatAsAtomicUnit=on
  Manipualtor pose in world frame : MATLAB Function  TreatAsAtomicUnit=on
  Math Function : Math  Operator=transpose  SaturateOnIntegerOverflow=on
  Mux1 : Mux
  Mux10 : Mux
  Mux2 : Mux  Inputs=3
  Mux5 : Mux
  Mux9 : Mux  Inputs=3
  Product1 : Product  Multiplication=Matrix(*)
  Product3 : Product  Multiplication=Matrix(*)
  Product4 : Product  Multiplication=Matrix(*)
  Quaternion Division1 : aerolibutil/Quaternion Division
  Quaternion Normalize : aerolibutil/Quaternion Normalize
  Spring Energy : Subsystem
  Wc1 : Outport
  tag scope: Manip1DampPower=global
  wires:
  Add2/1 -> Wc1/1
  Demux/1 -> Mux9/1
  Demux/2 -> Mux9/2
  Demux/3 -> Mux9/3
  Demux/4 -> Mux10/1
  Demux/5 -> Mux10/2
  Demux/6 -> Mux10/3
  Demux/7 -> Mux10/4
  MATLAB Function1/1(K) -> Product4/1
  Demux4/1 -> MATLAB Function1/3(eta)
  Add/1 -> Mux5/1
  Demux4/2 -> Mux5/2
  Demux4/3 -> Mux5/3
  Demux4/4 -> Mux5/4
  Mux5/1 -> Spring Energy/1(deltax), Product4/2
  Mux9/1 -> Add/1
  Manipualtor pose in world frame/1(pb1) -> Add/2
  Product4/1 -> Add2/1
  Mux10/1 -> Quaternion Division1/1
  Manipualtor pose in world frame/2(qb1) -> Quaternion Division1/2
  Add1/1 -> Product1/2, Product3/2
  dxb1/1 -> Add1/2
  Demux1/1 -> Mux2/1
  Demux1/2 -> Mux2/2
  Demux1/3 -> Mux2/3
  Demux1/4 -> Mux1/1
  Demux1/5 -> Mux1/2
  Demux1/6 -> Mux1/3
  Demux1/7 -> Mux1/4
  Mux2/1 -> Manipualtor pose in world frame/1(pb)
  Mux1/1 -> Manipualtor pose in world frame/2(qb)
  xb/1 -> Demux1/1
  Product1/1 -> Add2/2, Math Function/1
  Math Function/1 -> Product3/1
  Product3/1 -> [Manip1DampPower]
  Quaternion Division1/1 -> Quaternion Normalize/1
  Quaternion Normalize/1 -> Demux4/1
  x1/1 -> Demux/1
  dx1/1 -> Kinetic energy/1(dx), Add1/1
  [SETInternalDamping] -> Product1/1
  [SETInternalStiffness] -> Demux2/1
  Demux2/2 -> MATLAB Function1/2(kappas)
  Demux2/1 -> MATLAB Function1/1(ks)
  [SETrv] -> Manipualtor pose in world frame/3(rv)

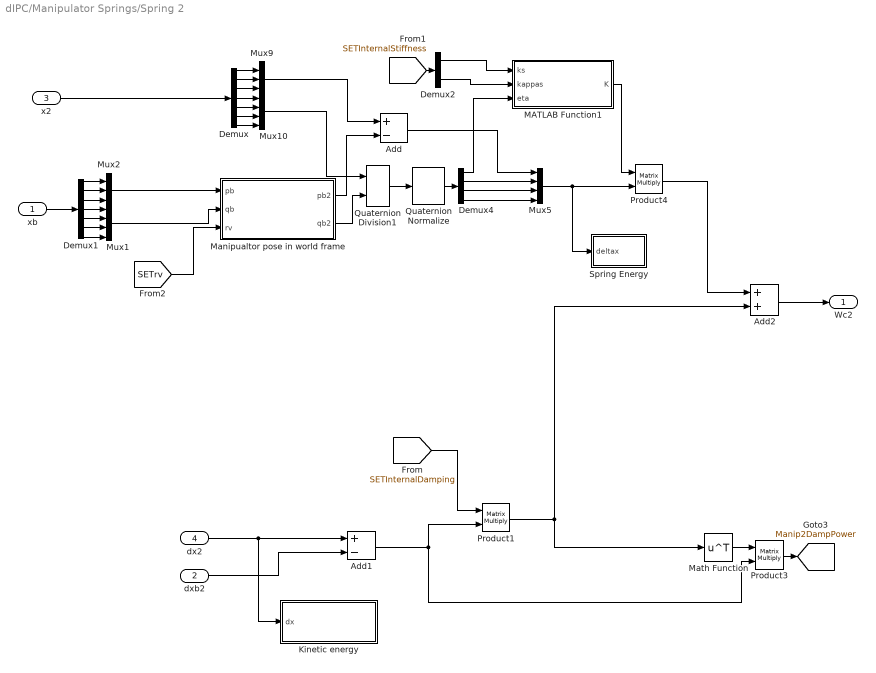
== system dIPC/Manipulator Springs/Spring 2 ==
  xb : Inport
  dxb2 : Inport  Port=2
  x2 : Inport  Port=3
  dx2 : Inport  Port=4
  Add : Sum  Inputs=+-
  Add1 : Sum  Inputs=+-
  Add2 : Sum
  Demux : Demux  Outputs=7
  Demux1 : Demux  Outputs=7
  Demux2 : Demux  Outputs=2
  Demux4 : Demux
  Kinetic energy : Subsystem
  MATLAB Function1 : MATLAB Function  TreatAsAtomicUnit=on
  Manipualtor pose in world frame : MATLAB Function  TreatAsAtomicUnit=on
  Math Function : Math  Operator=transpose  SaturateOnIntegerOverflow=on
  Mux1 : Mux
  Mux10 : Mux
  Mux2 : Mux  Inputs=3
  Mux5 : Mux
  Mux9 : Mux  Inputs=3
  Product1 : Product  Multiplication=Matrix(*)
  Product3 : Product  Multiplication=Matrix(*)
  Product4 : Product  Multiplication=Matrix(*)
  Quaternion Division1 : aerolibutil/Quaternion Division
  Quaternion Normalize : aerolibutil/Quaternion Normalize
  Spring Energy : Subsystem
  Wc2 : Outport
  tag scope: Manip2DampPower=global
  wires:
  Demux/1 -> Mux9/1
  Demux/2 -> Mux9/2
  Demux/3 -> Mux9/3
  Demux/4 -> Mux10/1
  Demux/5 -> Mux10/2
  Demux/6 -> Mux10/3
  Demux/7 -> Mux10/4
  MATLAB Function1/1(K) -> Product4/1
  Demux4/1 -> MATLAB Function1/3(eta)
  Add/1 -> Mux5/1
  Demux4/2 -> Mux5/2
  Demux4/3 -> Mux5/3
  Demux4/4 -> Mux5/4
  Quaternion Division1/1 -> Quaternion Normalize/1
  Mux5/1 -> Spring Energy/1(deltax), Product4/2
  Mux9/1 -> Add/1
  Manipualtor pose in world frame/1(pb2) -> Add/2
  Manipualtor pose in world frame/2(qb2) -> Quaternion Division1/2
  Mux10/1 -> Quaternion Division1/1
  Add2/1 -> Wc2/1
  Product4/1 -> Add2/1
  dxb2/1 -> Add1/2
  xb/1 -> Demux1/1
  Demux1/1 -> Mux2/1
  Demux1/2 -> Mux2/2
  Demux1/3 -> Mux2/3
  Demux1/4 -> Mux1/1
  Demux1/5 -> Mux1/2
  Demux1/6 -> Mux1/3
  Demux1/7 -> Mux1/4
  Mux2/1 -> Manipualtor pose in world frame/1(pb)
  Mux1/1 -> Manipualtor pose in world frame/2(qb)
  Add1/1 -> Product1/2, Product3/2
  Product1/1 -> Add2/2, Math Function/1
  Math Function/1 -> Product3/1
  Product3/1 -> [Manip2DampPower]
  Quaternion Normalize/1 -> Demux4/1
  x2/1 -> Demux/1
  dx2/1 -> Kinetic energy/1(dx), Add1/1
  [SETInternalStiffness] -> Demux2/1
  Demux2/2 -> MATLAB Function1/2(kappas)
  Demux2/1 -> MATLAB Function1/1(ks)
  [SETInternalDamping] -> Product1/1
  [SETrv] -> Manipualtor pose in world frame/3(rv)

== system dIPC/Manipulator motion/Angular Velocity to Quaternion ==
  omega_o : Inport
  Constant : Constant  Value=0
  Gain : Gain  Gain=0.5
  Integrator : Integrator  InitialCondition=[1; 0; 0; 0]
  Mux : Mux  Inputs=2
  Quaternion Multiplication : aerolibutil/Quaternion Multiplication
  Quaternion Normalize : aerolibutil/Quaternion Normalize
  Scope : Scope
      settings: ShowLegends=on  SaveName=ScopeData9
  q_o : Outport
  wires:
  omega_o/1 -> Gain/1
  Gain/1 -> Mux/2
  Constant/1 -> Mux/1
  Mux/1 -> Quaternion Multiplication/1
  Quaternion Multiplication/1 -> Integrator/1
  Integrator/1 -> Quaternion Normalize/1
  Quaternion Normalize/1 -> q_o/1, Scope/1, Quaternion Multiplication/2

== system dIPC/Object Spring1/Angular Velocity to Quaternion ==
  omega_o : Inport
  Constant : Constant  Value=0
  Gain : Gain  Gain=0.5
  Integrator : Integrator  InitialCondition=[1; 0; 0; 0]
  Mux : Mux  Inputs=2
  Quaternion Multiplication : aerolibutil/Quaternion Multiplication
  Scope : Scope
      settings: ShowLegends=on  SaveName=ScopeData9
  q_o : Outport
  wires:
  omega_o/1 -> Gain/1
  Gain/1 -> Mux/2
  Constant/1 -> Mux/1
  Quaternion Multiplication/1 -> Integrator/1
  Integrator/1 -> Quaternion Multiplication/2, q_o/1, Scope/1
  Mux/1 -> Quaternion Multiplication/1

== system dIPC/Object Spring1/Kinetic energy ==
  dx : Inport
  Constant : Constant  Value=blkdiag(0.5*mv*eye(3),0.5*jv*eye(3))
  Math Function : Math  Operator=transpose  SaturateOnIntegerOverflow=on
  Product : Product  Inputs=3  Multiplication=Matrix(*)
  tag scope: vObjectKineticEnergy=global
  wires:
  dx/1 -> Product/3, Math Function/1
  Math Function/1 -> Product/1
  Constant/1 -> Product/2
  Product/1 -> [vObjectKineticEnergy]

== system dIPC/Object Spring1/Spring Energy ==
  energy : Inport
  deltax : Inport  Port=2
  Constant : Constant  Commented=on  Value=blkdiag(0.5*kv*eye(3),2*kappav*eye(3))
  MATLAB Function1 : MATLAB Function  TreatAsAtomicUnit=on
  Math Function : Math  Operator=transpose  SaturateOnIntegerOverflow=on
  Product : Product  Inputs=3  Multiplication=Matrix(*)
  tag scope: vObjectSpringEnergy=global
  wires:
  deltax/1 -> Product/3, Math Function/1
  Math Function/1 -> Product/1
  Product/1 -> [vObjectSpringEnergy]
  energy/1 -> MATLAB Function1/1(energy)
  MATLAB Function1/1(K) -> Product/2

== system dIPC/Virtual Object Erhart/Angular Velocity to Quaternion ==
  omega_o : Inport
  Constant : Constant  Value=0
  Gain : Gain  Gain=0.5
  Integrator : Integrator  InitialCondition=[1; 0; 0; 0]
  Mux : Mux  Inputs=2
  Quaternion Multiplication : aerolibutil/Quaternion Multiplication
  Scope : Scope
      settings: ShowLegends=on  SaveName=ScopeData9
  q_o : Outport
  wires:
  omega_o/1 -> Gain/1
  Gain/1 -> Mux/2
  Constant/1 -> Mux/1
  Quaternion Multiplication/1 -> Integrator/1
  Integrator/1 -> Quaternion Multiplication/2, q_o/1, Scope/1
  Mux/1 -> Quaternion Multiplication/1

== system dIPC/Virtual Object Simulation/Angular Velocity to Quaternion ==
  omega_o : Inport
  Constant : Constant  Value=0
  Gain : Gain  Gain=0.5
  Integrator : Integrator  InitialCondition=[1; 0; 0; 0]
  Mux : Mux  Inputs=2
  Quaternion Multiplication : aerolibutil/Quaternion Multiplication
  Quaternion Normalize : aerolibutil/Quaternion Normalize
  q_o : Outport
  wires:
  omega_o/1 -> Gain/1
  Gain/1 -> Mux/2
  Constant/1 -> Mux/1
  Integrator/1 -> Quaternion Normalize/1
  Mux/1 -> Quaternion Multiplication/1
  Quaternion Multiplication/1 -> Integrator/1
  Quaternion Normalize/1 -> q_o/1, Quaternion Multiplication/2

== system dIPC/Manipulator Springs/Spring 1/Kinetic energy ==
  dx : Inport
  Constant : Constant  Value=blkdiag(0.5*m1*eye(3),0.5*j1*eye(3))
  Math Function : Math  Operator=transpose  SaturateOnIntegerOverflow=on
  Product : Product  Inputs=3  Multiplication=Matrix(*)
  tag scope: Manip1KineticEnergy=global
  wires:
  dx/1 -> Product/3, Math Function/1
  Math Function/1 -> Product/1
  Constant/1 -> Product/2
  Product/1 -> [Manip1KineticEnergy]

== system dIPC/Manipulator Springs/Spring 1/Spring Energy ==
  deltax : Inport
  Constant : Constant  Value=blkdiag(0.5*ks*eye(3),2*kappas*eye(3))
  Math Function : Math  Operator=transpose  SaturateOnIntegerOverflow=on
  Product : Product  Inputs=3  Multiplication=Matrix(*)
  tag scope: Manip1SpringEnergy=global
  wires:
  deltax/1 -> Product/3, Math Function/1
  Math Function/1 -> Product/1
  Constant/1 -> Product/2
  Product/1 -> [Manip1SpringEnergy]

== system dIPC/Manipulator Springs/Spring 2/Kinetic energy ==
  dx : Inport
  Constant : Constant  Value=blkdiag(0.5*m2*eye(3),0.5*j2*eye(3))
  Math Function : Math  Operator=transpose  SaturateOnIntegerOverflow=on
  Product : Product  Inputs=3  Multiplication=Matrix(*)
  tag scope: Manip2KineticEnergy=global
  wires:
  dx/1 -> Product/3, Math Function/1
  Math Function/1 -> Product/1
  Constant/1 -> Product/2
  Product/1 -> [Manip2KineticEnergy]

== system dIPC/Manipulator Springs/Spring 2/Spring Energy ==
  deltax : Inport
  Constant : Constant  Value=blkdiag(0.5*ks*eye(3),2*kappas*eye(3))
  Math Function : Math  Operator=transpose  SaturateOnIntegerOverflow=on
  Product : Product  Inputs=3  Multiplication=Matrix(*)
  tag scope: Manip2SpringEnergy=global
  wires:
  deltax/1 -> Product/3, Math Function/1
  Math Function/1 -> Product/1
  Constant/1 -> Product/2
  Product/1 -> [Manip2SpringEnergy]

== matlab function dIPC/Manipulator Springs/Spring 1/Manipualtor pose in world frame ==
  data: pb input; qb input size=4; pb1 output; rv input; qb1 output
function [pb1,qb1]= manipulatorpose(pb,qb,rv)

pb1 = pb + quatrot(qb,rv(1:3));
qb1 = qb;

== matlab function dIPC/Manipulator Springs/Spring 2/Manipualtor pose in world frame ==
  data: pb input; qb input size=4; pb2 output; rv input; qb2 output
function [pb2,qb2]= manipulatorpose(pb,qb,rv)

pb2 = pb + quatrot(qb,rv(4:6));
qb2 = qb;

== matlab function dIPC/Object Spring1/MATLAB Function1 ==
  data: energy input size=1; kv input; kappav input; eta input; K output
function K = stiffness(energy, kv,kappav, eta)
if energy>10
    energy=10;
%elseif energy<0
 %    energy=0;
end
K = blkdiag(kv*energy/10*eye(3),2*eta*kappav*energy/10*eye(3));
%K = blkdiag(kv*eye(3),2*eta*kappav*eye(3));

== matlab function dIPC/Interaction dynamics1/MATLAB Function ==
  data: r input; A output; x input
function A = ConstraintMatrix(r,x)
A = [-eye(3) skew_sm(quatrot(x(4:7),r(1:3))) eye(3) zeros(3,9);
        zeros(3) -eye(3) zeros(3) eye(3) zeros(3,6);
        -eye(3) skew_sm(quatrot(x(4:7),r(4:6))) zeros(3,6) eye(3) zeros(3);
        zeros(3) -eye(3) zeros(3,9) eye(3)];

== matlab function dIPC/Interaction dynamics1/Centripetal Force ==
  data: dx input; b output; x input; r input
function b = centripetalforce(dx,x, r)
b = [skew_sm(dx(4:6))*skew_sm(dx(4:6))*quatrot(x(4:7),r(1:3));
     zeros(3,1);
     skew_sm(dx(4:6))*skew_sm(dx(4:6))*quatrot(x(4:7),r(4:6));
     zeros(3,1)];

== matlab function dIPC/Interaction dynamics1/Coriolis Force ==
  data: dx input; hcoriolis output; j0 parameter; m0 parameter
function hcoriolis = CoriolisForce(dx,j0,m0)
hcoriolis = [m0*skew_sm(dx(4:6))*dx(1:3);
        j0*skew_sm(dx(4:6))*dx(4:6)];

== matlab function dIPC/Manipulator Springs/Spring 1/MATLAB Function1 ==
  data: K output; ks input; kappas input; eta input
function K = stiffness(ks,kappas, eta)
K = blkdiag(ks*eye(3),2*eta*kappas*eye(3));

== matlab function dIPC/Manipulator Springs/Spring 2/MATLAB Function1 ==
  data: K output; ks input; kappas input; eta input
function K = stiffness(ks, kappas, eta)
K = blkdiag(ks*eye(3),2*eta*kappas*eye(3));

== matlab function dIPC/Virtual Object Simulation/Grasp Matrix ==
  data: G output; x input; rv input
function G = GraspMatrix(x, rv)
G = [eye(3) zeros(3) eye(3) zeros(3);
    skew_sm(quatrot(x(4:7),rv(1:3))) eye(3) skew_sm(quatrot(x(4:7),rv(4:6))) eye(3)];

== matlab function dIPC/Virtual Object Erhart/Centripetal Force ==
  data: dx input size=6; b output; rv parameter; x input size=7
function b = centripetalforce(dx,rv,x)
b = [skew_sm(dx(4:6))*skew_sm(dx(4:6))*quatrot(x(4:7),rv(1:3));
     zeros(3,1);
     skew_sm(dx(4:6))*skew_sm(dx(4:6))*quatrot(x(4:7),rv(4:6));
     zeros(3,1);
     skew_sm(dx(4:6))*skew_sm(dx(4:6))*quatrot(x(4:7),rv(7:9));
     zeros(3,1);
     skew_sm(dx(4:6))*skew_sm(dx(4:6))*quatrot(x(4:7),rv(10:12));
     zeros(3,1)];

== matlab function dIPC/Virtual Object Erhart/Coriolis Force ==
  data: dx input; hcoriolis output; j0 parameter; m0 parameter
function hcoriolis = CoriolisForce(dx,j0,m0)
hcoriolis = [m0*skew_sm(dx(4:6))*dx(1:3);
        j0*skew_sm(dx(4:6))*dx(4:6)];

== matlab function dIPC/Virtual Object Erhart/MATLAB Function ==
  data: rv parameter; A output; x input
function A = ConstraintMatrix(rv,x)
A = [-eye(3) skew_sm(quatrot(x(4:7),rv(1:3))) eye(3) zeros(3,21);
        zeros(3) -eye(3) zeros(3) eye(3) zeros(3,18);
        -eye(3) skew_sm(quatrot(x(4:7),rv(4:6))) zeros(3,6) eye(3) zeros(3,15);
        zeros(3) -eye(3) zeros(3,9) eye(3) zeros(3,12);
        -eye(3) skew_sm(quatrot(x(4:7),rv(7:9))) zeros(3,12) eye(3) zeros(3,9);
        zeros(3) -eye(3) zeros(3,15) eye(3) zeros(3,6);
        -eye(3) skew_sm(quatrot(x(4:7),rv(10:12))) zeros(3,18) eye(3) zeros(3);
        zeros(3) -eye(3) zeros(3,21) eye(3)];

== matlab function dIPC/Manipulator Springs/Grasp Matrix ==
  data: G output; x input; rv input
function G = GraspMatrix(x, rv)
G = [eye(3) zeros(3) eye(3) zeros(3);
    skew_sm(quatrot(x(4:7),rv(1:3))) eye(3) skew_sm(quatrot(x(4:7),rv(4:6))) eye(3)];

== matlab function dIPC/Object Spring1/Spring Energy/MATLAB Function1 ==
  data: K output; kv parameter; kappav parameter; energy input
function K = stiffness(kv,kappav,energy)
if energy>10
    energy=10;
% elseif energy<1
%     energy=1;
end
K = blkdiag(0.5*kv*energy/10*eye(3),2*kappav*energy/10*eye(3));
%K = blkdiag(0.5*kv*eye(3),2*kappav*eye(3));

== matlab function dIPC/Object Spring1/MATLAB Function2 ==
  data: energy input size=1; dv input; D output; deltav input
function D = vardamping(energy, dv,deltav)
if energy>10
    energy=10;
%elseif energy<0.5
%    energy=0.5;
end
D = blkdiag(dv*energy/10*eye(3),deltav*energy/10*eye(3));
%D = blkdiag(dv/100*energy*eye(3),deltav/100*energy*eye(3));

== matlab function dIPC/Manipulator dynamics/Reduced Constraint Matrix ==
  data: r input; Ared output; x input
function Ared = ReducedConstraintMAtrix(r,x)
Ared = [-eye(3) skew_sm(quatrot(x(4:7),r(4:6)-r(1:3))) eye(3) zeros(3);
        zeros(3) -eye(3) zeros(3) eye(3)];

== matlab function dIPC/Manipulator dynamics/Centripal Force ==
  data: r input; x input; bred output; dx input
function bred = ReducedCentripetalvector(r,x,dx)
bred = [skew_sm(dx(4:6))*skew_sm(dx(4:6))*quatrot(x(4:7),(r(4:6)-r(1:3)));
        zeros(3,1)];

== matlab function dIPC/Manipulator motion/Grasp Matrix ==
  data: G output; x input; r input
function G = GraspMatrix(x, r)
G = [eye(3) zeros(3) eye(3) zeros(3);
    skew_sm(quatrot(x(4:7),r(1:3))) eye(3) skew_sm(quatrot(x(4:7),r(4:6))) eye(3)];

== matlab function dIPC/Manipulator motion/Manipualtor pose in world frame ==
  data: p_o input; q_o input size=4; x output; r input
function x = manipulatorpose(p_o,q_o,r)

x = [p_o + quatrot(q_o,r(1:3));
        q_o;
        p_o + quatrot(q_o,r(4:6));
        q_o];

== matlab function dIPC/Manipulator dynamics/World to Object Frame ==
  data: hw input; x input; h_int output
function h_int = inertial2objectFrame(hw,x)

h_int = [quatrot(quatconj(x(4:7)')',hw(1:3));
         hw(4:6);%quatrot(quatconj(x(4:7)')',hw(4:6));
         quatrot(quatconj(x(4:7)')',hw(7:9));
         hw(10:12)];%quatrot(quatconj(x(4:7)')',hw(10:12));
